simulink model "sendWfmToPWM"  (R2026a)
settings: Solver=FixedStepAuto  EnableMultiTasking=on
model workspace: external: MAT-File C:\Users\LENOVO\OneDrive\Documents\tfg\biosignalSim\storedECGSignal.mat (data not in the file)
values from neighbouring files (symbols this model uses):
  dt = t_(2) - t_(1)    [DutyToSquare.m]    (also in modelVariables.mat = 0.001; storedECGSignal.mat = 0.001)
  nsamples = 15022    [storedECGSignal.mat]
  wfm = [wfm, wfm_interval]    [DutyArrayToPWM.m]    (also in DutyToSquare.m = [wfm, 0]; addBLW.m = wfm_; generateECGPeriod.m = zeros(1,size(t,2)); generateNCycles.m = wfm_b)
libraries: simulink x1, stm32f4xxblockslib x1
settings Model: STM32="{\"PWMOutput\":{\"ID\":\"162\"}}"  Creator=LENOVO  LastModifiedBy=LENOVO
settings OptimizationCC: MaxStackSize=512
settings HardwareCC: ProdLargestAtomicInteger=Long  ProdLargestAtomicFloat=Double  ProdHWDeviceType=ARM Compatible->ARM Cortex-M
settings RTWCC: SystemTargetFile=ert.tlc  HardwareBoard=STM32F4xx Based  TLCOptions=-aInlineSetEventsForThisBaseRateFcn=TLC_FALSE -aSuppressMultiTaskScheduler=TLC_FALSE -aRateBasedStepFcn=1  Toolchain=GNU Tools for STM32  BuildConfiguration=Faster Runs  Description=Embedded Coder
settings ERTTargetCC: ExtModeTransport=3.0  ExtModeStaticAllocSize=2048.0  CodeReplacementLibrary=ARM Cortex-M  SupportContinuousTime=on

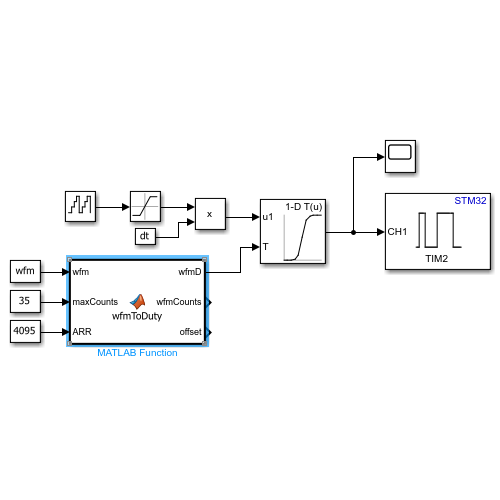
[thumbnail: Simulink's stored preview of the top-level diagram]
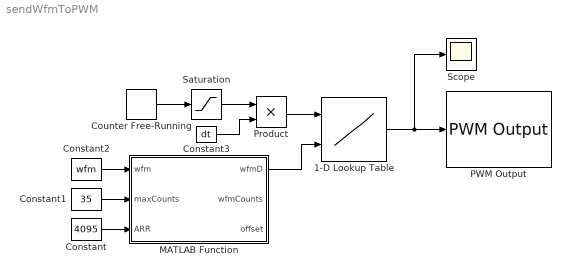
== system sendWfmToPWM ==
  1-D Lookup Table : Lookup_n-D  NumberOfTableDimensions=1  BreakpointsForDimension1=t  BreakpointsForDimension1DataTypeStr=double  TableSource=Input port  Table=sin(0.005*[1:1:nsamples])  TableDataTypeStr=double  IntermediateResultsDataTypeStr=double  ExtrapMethod=Clip  InternalRulePriority=Speed  OutDataTypeStr=double  RndMeth=Simplest  FractionDataTypeStr=double
      settings: InputPortMap=u0,p221
  Constant : Constant  Value=4095
  Constant1 : Constant  Value=35
  Constant2 : Constant  Value=wfm
  Constant3 : Constant  Value=dt
  Counter Free-Running : simulink/Sources/Counter Free-Running  NumBits=17  tsamp=dt
  MATLAB Function : MATLAB Function  TreatAsAtomicUnit=on
  PWM Output : stm32f4xxblockslib/PWM Output  ProcessorFamily=STM32F4  TimerModule=TIM2  DutycycleUnits=Percentage  EnableChannel1=on  EnableCaptureCompare1Input=off  EnableCaptureCompare1ComplementaryInput=off  EnableOutputCompare1ModeInput=off  EnableChannel2=off  EnableCaptureCompare2Input=off  EnableCaptureCompare2ComplementaryInput=off  EnableOutputCompare2ModeInput=off  EnableChannel3=off  EnableCaptureCompare3Input=off  EnableCaptureCompare3ComplementaryInput=off  EnableOutputCompare3ModeInput=off  EnableChannel4=off  EnableCaptureCompare4Input=off  EnableCaptureCompare4ComplementaryInput=off  EnableOutputCompare4ModeInput=off  EnableChannel5=off  EnableCaptureCompare5Input=off  EnableOutputCompare5ModeInput=off  EnableChannel6=off  EnableCaptureCompare6Input=off  EnableOutputCompare6ModeInput=off  EnableCounterInput=off  EnableMainOutputInput=off  EnableFrequencyInput=off  SetRCAfterCE=off  OutputDirection=off  OutputMainOutputEnableStatus=off  SampleTime=0.1  EnableSimPort=off  EnableUpdateEvent=off  EnableCaptureCompare1Event=off  EnableCaptureCompare2Event=off  EnableCaptureCompare3Event=off  EnableCaptureCompare4Event=off  EnableTriggerEvent=off  EnableBreakEvent=off  EnableBreakEvent2=off  hoistedMaskSrc=ECSoC/ECSimCodegen/PWM Output
  Product : Product
  Saturation : Saturate  UpperLimit=nsamples  LowerLimit=0
  Scope : Scope
      settings: ActiveDisplayYMinimum=-0.10683195796938623  ActiveDisplayYMaximum=0.96151008678040761
  wires:
  Counter Free-Running/1 -> Saturation/1
  Constant/1 -> MATLAB Function/3(ARR)
  Constant2/1 -> MATLAB Function/1(wfm)
  1-D Lookup Table/1 -> Scope/1, PWM Output/1
  Constant1/1 -> MATLAB Function/2(maxCounts)
  MATLAB Function/1(wfmD) -> 1-D Lookup Table/2
  Product/1 -> 1-D Lookup Table/1
  Saturation/1 -> Product/1
  Constant3/1 -> Product/2

== matlab function sendWfmToPWM/MATLAB Function ==
  data: wfm input; wfmD output; wfmCounts output; maxCounts input; ARR input; offset output
function [wfmD, wfmCounts, offset] = wfmToDuty(wfm,maxCounts,ARR)

    %%% Turns the input waveform into a series of PWM duty cycles (%)
    %%% maxCounts is the number of counts needed to get the maximum wfm value (could be ARR or less, for example if your pin is 0-5V but if you need a maximum output voltage of less than 5V, it might interest you to set a lower maxCount value)
    
    if min(wfm) < 0
        %%% Removes negative values
        offset = abs(min(wfm));
    else
        offset = 0;
    end

    wfm = wfm + offset;
    wfmCounts = wfm * (maxCounts/max(wfm));
    wfmD = (wfmCounts/ARR)*100;
    
end
